simulink model "soac_mc_test"  (R2018b)
settings: Solver=FixedStepAuto  StartTime=0.0  StopTime=60  FixedStep=soac_params.sample_time_s  RelTol=1e-3
values from neighbouring files (symbols this model uses):
  GPS_epoch = sim_params.environment.sgp4.gps_time    [soac_mc_test_init.m]
  hw_in = horzcat(eye(3),zeros(3,1)) * hw0    [soac_mc_test_init.m]
  omega_cmd = [ 0.0; 0.0; 0.0 ]    [soac_mc_test_init.m]
  omega_in = zeros(3,1) + var_w.*randn(3,1)    [soac_mc_test_init.m]
  quat_cmd = [ 1.0; 0.0; 0.0; 0.0 ]    [soac_mc_test_init.m]
  sI_unit = [ 1.0; 0.0; 0.0 ]    [soac_mc_test_init.m]
undefined symbols (not defined in the file or in its folder): DiscIntNeverNeededParam, fsw_params, GPS_time_lib, sim_params, soac_params
libraries: aerolibutil x3, simulink x2, vrlib x1, quat_degerr_check x1, quat_degerr_lib x1, dynamics_lib x1, soac_interface_lib x1
settings Model: Creator=taylorreynolds  LastModifiedBy=Taylor
settings DebuggingCC: SingleTaskRateTransMsg=error
settings SFSimCC: SimUseLocalCustomCode=off
settings RTWCC: GenerateReport=on  RTWUseLocalCustomCode=off  LaunchReport=on
settings CodeAppCC: StateflowObjectComments=on

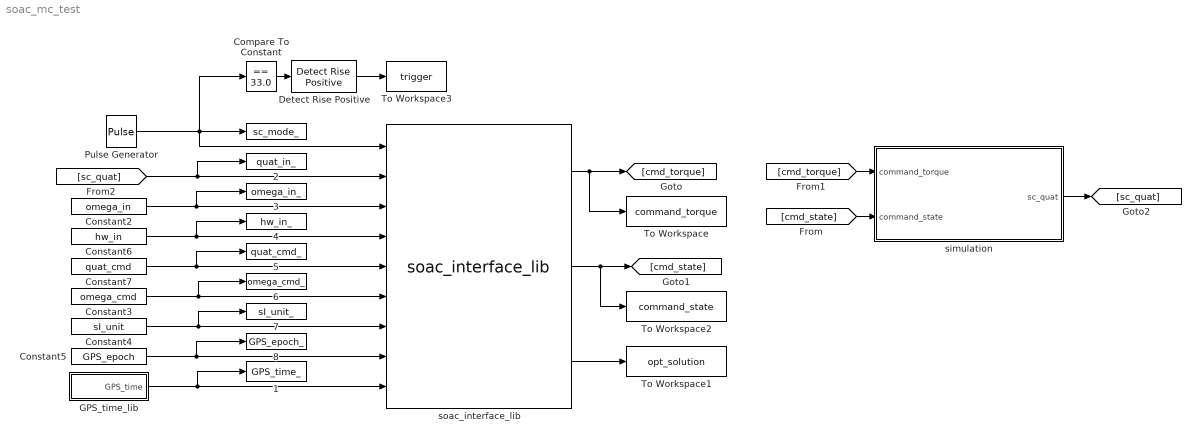
== system soac_mc_test ==
  " " : ToWorkspace  VariableName=sc_mode_  SaveFormat=Timeseries  SampleTime=-1
  " 1" : ToWorkspace  VariableName=GPS_time_  SaveFormat=Timeseries  SampleTime=-1
  " 2" : ToWorkspace  VariableName=quat_in_  SaveFormat=Timeseries  SampleTime=-1
  " 3" : ToWorkspace  VariableName=omega_in_  SaveFormat=Timeseries  SampleTime=-1
  " 4" : ToWorkspace  VariableName=hw_in_  SaveFormat=Timeseries  SampleTime=-1
  " 5" : ToWorkspace  VariableName=quat_cmd_  SaveFormat=Timeseries  SampleTime=-1
  " 6" : ToWorkspace  VariableName=omega_cmd_  SaveFormat=Timeseries  SampleTime=-1
  " 7" : ToWorkspace  VariableName=sI_unit_  SaveFormat=Timeseries  SampleTime=-1
  " 8" : ToWorkspace  VariableName=GPS_epoch_  SaveFormat=Timeseries  SampleTime=-1
  Compare To Constant : simulink/Logic and Bit Operations/Compare To Constant  relop===  const=33.0  OutDataTypeStr=boolean
  Constant2 : Constant  Value=omega_in  SampleTime=soac_params.sample_time_s
  Constant3 : Constant  Value=omega_cmd  SampleTime=soac_params.sample_time_s
  Constant4 : Constant  Value=sI_unit  SampleTime=soac_params.sample_time_s
  Constant5 : Constant  Value=GPS_epoch  SampleTime=soac_params.sample_time_s
  Constant6 : Constant  Value=hw_in  SampleTime=soac_params.sample_time_s
  Constant7 : Constant  Value=quat_cmd  SampleTime=soac_params.sample_time_s
  Detect Rise Positive : simulink/Logic and Bit Operations/Detect Rise Positive  vinit=0  OutDataTypeStr=boolean
  GPS_time_lib : Subsystem  AncestorBlock=GPS_time_lib/GPS_time_lib
  Pulse Generator : DiscretePulseGenerator  PulseType=Time based  Amplitude=33  Period=100  PulseWidth=5
  To Workspace : ToWorkspace  VariableName=command_torque  SampleTime=-1
  To Workspace1 : ToWorkspace  VariableName=opt_solution  SaveFormat=Timeseries  SampleTime=-1
  To Workspace2 : ToWorkspace  VariableName=command_state  SampleTime=-1
  To Workspace3 : ToWorkspace  VariableName=trigger  SampleTime=-1
  simulation : Subsystem
  soac_interface_lib : soac_interface_lib/soac_interface_lib  SystemSampleTime=-1
  wires:
  GPS_time_lib/1(GPS_time) -> soac_interface_lib/9, " 1"/1
  Constant5/1 -> soac_interface_lib/8, " 8"/1
  soac_interface_lib/1 -> [cmd_torque], To Workspace/1
  soac_interface_lib/3 -> To Workspace1/1
  Constant6/1 -> soac_interface_lib/4, " 4"/1
  Constant7/1 -> soac_interface_lib/5, " 5"/1
  Constant4/1 -> soac_interface_lib/7, " 7"/1
  Constant2/1 -> soac_interface_lib/3, " 3"/1
  [sc_quat] -> soac_interface_lib/2, " 2"/1
  Pulse Generator/1 -> Compare To Constant/1, soac_interface_lib/1, " "/1
  soac_interface_lib/2 -> [cmd_state], To Workspace2/1
  [cmd_torque] -> simulation/1(command_torque)
  [cmd_state] -> simulation/2("command_state ")
  Constant3/1 -> soac_interface_lib/6, " 6"/1
  simulation/1(sc_quat) -> [sc_quat]
  Compare To Constant/1 -> Detect Rise Positive/1
  Detect Rise Positive/1 -> To Workspace3/1

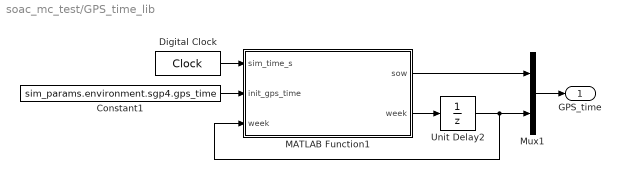
== system soac_mc_test/GPS_time_lib ==
  Constant1 : Constant  Value=sim_params.environment.sgp4.gps_time  SampleTime=soac_params.sample_time_s
  Digital Clock : DigitalClock  SampleTime=soac_params.sample_time_s
  MATLAB Function1 : MATLAB Function  TreatAsAtomicUnit=on
  Mux1 : Mux  Inputs=2
  Unit Delay2 : UnitDelay  InitialCondition=sim_params.environment.sgp4.gps_week_init  SampleTime=-1
  GPS_time : Outport
  wires:
  Digital Clock/1 -> MATLAB Function1/1(sim_time_s)
  Constant1/1 -> MATLAB Function1/2(init_gps_time)
  MATLAB Function1/2(week) -> Unit Delay2/1
  Unit Delay2/1 -> MATLAB Function1/3("week "), Mux1/2
  MATLAB Function1/1(sow) -> Mux1/1
  Mux1/1 -> GPS_time/1

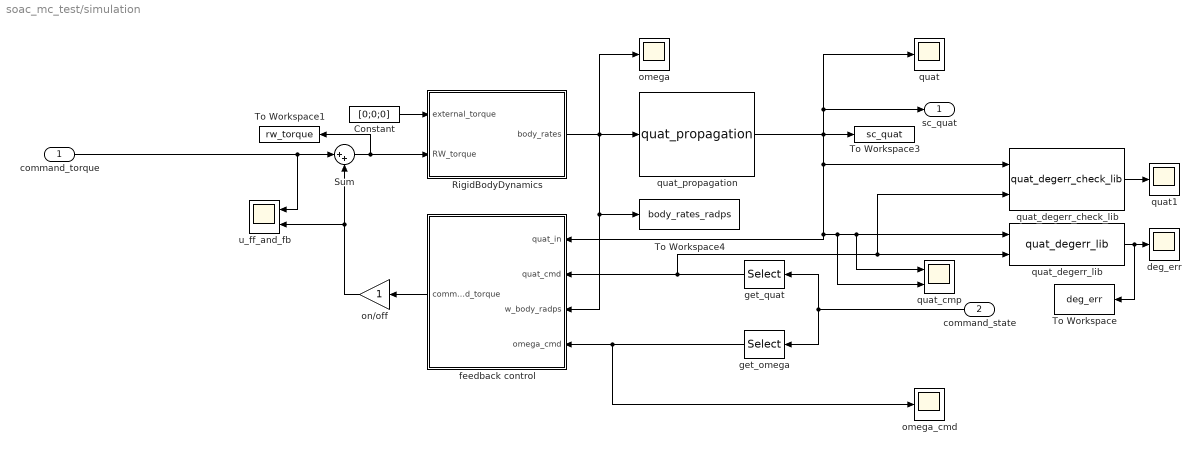
== system soac_mc_test/simulation ==
  command_torque : Inport
  "command_state " : Inport  Port=2
  Constant : Constant  Value=[0;0;0]
  RigidBodyDynamics : Subsystem  AncestorBlock=dynamics_lib/Dynamics/RigidBodyDynamics
  Sum : Sum  Inputs=|++
  To Workspace : ToWorkspace  VariableName=deg_err  SampleTime=-1
  To Workspace1 : ToWorkspace  VariableName=rw_torque  SampleTime=-1
  To Workspace3 : ToWorkspace  VariableName=sc_quat  SampleTime=-1
  To Workspace4 : ToWorkspace  VariableName=body_rates_radps  SampleTime=-1
  deg_err : Scope
  feedback control : Subsystem  AncestorBlock=pd_control_lib/PD Control
  get_omega : Selector  InputPortWidth=10  IndexOptions=Index vector (dialog)  Indices=[5 6 7]  OutputSizes=1
  get_quat : Selector  InputPortWidth=10  IndexOptions=Index vector (dialog)  Indices=[1 2 3 4]  OutputSizes=1
  omega : Scope
  omega_cmd : Scope
  on/off : Gain
  quat : Scope
  quat1 : Scope
  quat_cmp : Scope  NumInputPorts=2
  quat_degerr_check_lib : quat_degerr_check/quat_degerr_check_lib  point_tol=1
  quat_degerr_lib : quat_degerr_lib/quat_degerr_lib  SystemSampleTime=-1
  quat_propagation : dynamics_lib/Dynamics/quat_propagation  SystemSampleTime=-1
  u_ff_and_fb : Scope  NumInputPorts=2
  sc_quat : Outport
  wires:
  RigidBodyDynamics/1(body_rates) -> omega/1, feedback control/3(w_body_radps), To Workspace4/1, quat_propagation/1
  Constant/1 -> RigidBodyDynamics/1(external_torque)
  get_quat/1 -> quat_degerr_lib/2, quat_degerr_check_lib/2, feedback control/2(quat_cmd)
  quat_degerr_check_lib/1 -> quat1/1
  quat_propagation/1 -> feedback control/1(quat_in), quat_cmp/2, quat_cmp/1, quat_degerr_lib/1, quat_degerr_check_lib/1, To Workspace3/1, sc_quat/1, quat/1
  "command_state "/1 -> get_quat/1, get_omega/1
  Sum/1 -> To Workspace1/1, RigidBodyDynamics/2(RW_torque)
  get_omega/1 -> omega_cmd/1, feedback control/4(omega_cmd)
  command_torque/1 -> u_ff_and_fb/1, Sum/1
  feedback control/1(command_torque) -> on/off/1
  on/off/1 -> u_ff_and_fb/2, Sum/2
  quat_degerr_lib/1 -> To Workspace/1, deg_err/1

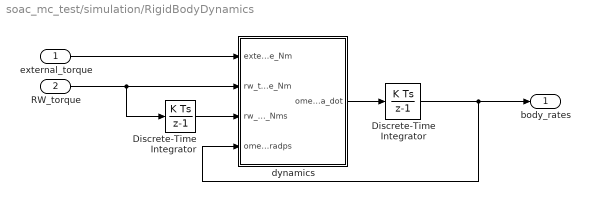
== system soac_mc_test/simulation/RigidBodyDynamics ==
  external_torque : Inport
  RW_torque : Inport  Port=2
  Discrete-Time Integrator : DiscreteIntegrator  InitialCondition=sim_params.actuators.reaction_wheel.ic.body_momentum  SampleTime=-1  ICPrevOutput=DiscIntNeverNeededParam  ICPrevScaledInput=DiscIntNeverNeededParam
  "Discrete-Time Integrator " : DiscreteIntegrator  InitialCondition=sim_params.dynamics.ic.rate_init  SampleTime=-1  ICPrevOutput=DiscIntNeverNeededParam  ICPrevScaledInput=DiscIntNeverNeededParam
  dynamics : Subsystem
  body_rates : Outport
  wires:
  RW_torque/1 -> dynamics/2(rw_torque_Nm), Discrete-Time Integrator/1
  Discrete-Time Integrator/1 -> dynamics/3(rw_momentum_Nms)
  "Discrete-Time Integrator "/1 -> body_rates/1, dynamics/4(omega_radps)
  external_torque/1 -> dynamics/1(external_torque_Nm)
  dynamics/1(omega_dot) -> "Discrete-Time Integrator "/1

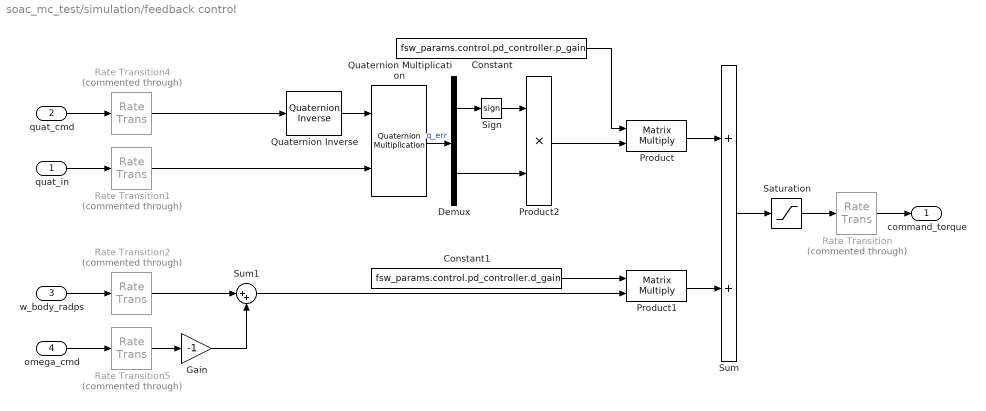
== system soac_mc_test/simulation/feedback control ==
  quat_in : Inport
  quat_cmd : Inport  Port=2
  w_body_radps : Inport  Port=3
  omega_cmd : Inport  Port=4
  Constant : Constant  Value=fsw_params.control.pd_controller.p_gain
  Constant1 : Constant  Value=fsw_params.control.pd_controller.d_gain
  Demux : Demux  Outputs=[1 3]
  Gain : Gain  Gain=-1
  Product : Product  Multiplication=Matrix(*)
  Product1 : Product  Multiplication=Matrix(*)
  Product2 : Product
  Quaternion Inverse : aerolibutil/Quaternion Inverse
      settings: SourceProductName=Aerospace Blockset
  Quaternion Multiplication : aerolibutil/Quaternion Multiplication
  Rate Transition : RateTransition  Commented=through  InitialCondition=fsw_params.control.pd_controller.ic.rt_command_torque
  Rate Transition1 : RateTransition  Commented=through  InitialCondition=fsw_params.control.pd_controller.ic.rt_quat_in  OutPortSampleTime=fsw_params.control.pd_controller.sample_time_s
  Rate Transition2 : RateTransition  Commented=through  InitialCondition=fsw_params.control.pd_controller.ic.rt_w_body_radps  OutPortSampleTime=fsw_params.control.pd_controller.sample_time_s
  Rate Transition4 : RateTransition  Commented=through  InitialCondition=fsw_params.control.pd_controller.ic.rt_quat_in  OutPortSampleTime=fsw_params.control.pd_controller.sample_time_s
  Rate Transition5 : RateTransition  Commented=through  InitialCondition=fsw_params.control.pd_controller.ic.rt_w_body_radps  OutPortSampleTime=fsw_params.control.pd_controller.sample_time_s
  Saturation : Saturate  UpperLimit=fsw_params.bus.max_torque  LowerLimit=-fsw_params.bus.max_torque
  Sign : Signum
  Sum : Sum
  Sum1 : Sum  Inputs=|++
  command_torque : Outport
  wires:
  Product2/1 -> Product/2
  Sign/1 -> Product2/1
  Sum1/1 -> Product1/2
  Gain/1 -> Sum1/2
  Rate Transition5/1 -> Gain/1
  Rate Transition2/1 -> Sum1/1
  omega_cmd/1 -> Rate Transition5/1
  Rate Transition4/1 -> Quaternion Inverse/1
  Rate Transition1/1 -> Quaternion Multiplication/2
  Rate Transition/1 -> command_torque/1
  Sum/1 -> Saturation/1
  Product1/1 -> Sum/2
  Product/1 -> Sum/1
  Demux/2 -> Product2/2
  w_body_radps/1 -> Rate Transition2/1
  Demux/1 -> Sign/1
  Quaternion Multiplication/1 -> Demux/1  "q_err"
  quat_in/1 -> Rate Transition1/1
  Quaternion Inverse/1 -> Quaternion Multiplication/1
  quat_cmd/1 -> Rate Transition4/1
  Constant/1 -> Product/1
  Constant1/1 -> Product1/1
  Saturation/1 -> Rate Transition/1

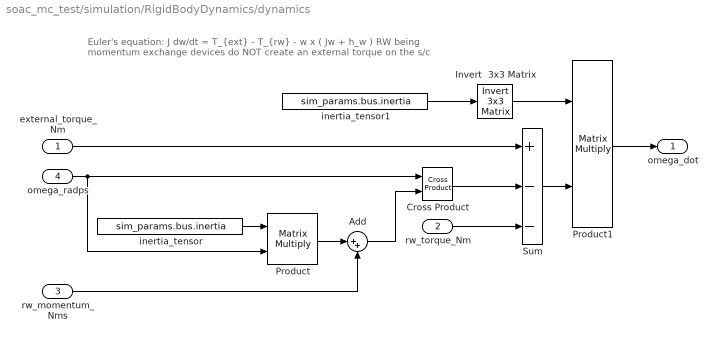
== system soac_mc_test/simulation/RigidBodyDynamics/dynamics ==
  note: Euler's equation: J dw/dt = T_{ext} - T_{rw} - w x ( Jw + h_w )
      |
      | RW being momentum exchange devices do NOT create
      | an external torque on the s/c
  external_torque_Nm : Inport
  rw_torque_Nm : Inport  Port=2
  rw_momentum_Nms : Inport  Port=3
  omega_radps : Inport  Port=4
  Add : Sum  Inputs=|++
  Cross Product : vrlib/Utilities/Cross Product
      settings: SourceProductBaseCode=VR
  Invert  3x3 Matrix : aerolibutil/Invert  3x3 Matrix
  Product : Product  Multiplication=Matrix(*)  RndMeth=Zero
  Product1 : Product  Multiplication=Matrix(*)  RndMeth=Zero
  Sum : Sum  Inputs=+--
  inertia_tensor : Constant  Value=sim_params.bus.inertia  SampleTime=-1
  inertia_tensor1 : Constant  Value=sim_params.bus.inertia  SampleTime=-1
  omega_dot : Outport
  wires:
  rw_torque_Nm/1 -> Sum/3
  Add/1 -> Cross Product/2
  rw_momentum_Nms/1 -> Add/2
  Product/1 -> Add/1
  Cross Product/1 -> Sum/2
  inertia_tensor1/1 -> Invert  3x3 Matrix/1
  Invert  3x3 Matrix/1 -> Product1/1
  Product1/1 -> omega_dot/1
  Sum/1 -> Product1/2
  inertia_tensor/1 -> Product/1
  omega_radps/1 -> Cross Product/1, Product/2
  external_torque_Nm/1 -> Sum/1

== matlab function soac_mc_test/GPS_time_lib/MATLAB Function1 ==
  data: sim_time_s input; sow output; init_gps_time input; week input; week output
function [sow, week] = gps_clock(sim_time_s, init_gps_time, week)
% ----------------------------------------------------------------------- %
% UW HuskySat-1, ADCS Subsystem
%
% GPS clock for the SIM.
% ----------------------------------------------------------------------- %

% Constants
sec_in_week = 604800;


init_sow    = init_gps_time(1);
sow         = mod(init_sow + sim_time_s, sec_in_week);

% Handle roll overs
if sow == sec_in_week
    week = week + 1;
end

end
